simulink model "mrefrobotarm_modified_previous_y_previous_u_previous_ref"  (R2018b)
settings: Solver=FixedStepAuto  StartTime=0.0  StopTime=10  RelTol=1e-3  AbsTol=1e-6
undefined symbols (not defined in the file or in its folder): options, sfunxy2
libraries: neural x949, simulink x1
(part 18 of 31)

== system mrefrobotarm_modified_previous_y_previous_u_previous_ref/const_51traces_100/Layer 2/Delays 1 ==
  "p{2}" : Inport  PortDimensions=100
      mask Display: e = 0.06;c1 = [120 230 180]/255;c2 = ([120 230 180]+0)/(256+128);c3 = ([120 230 180]+128)/(256+128);patch([0 1 1 0],[0 0 1 1],c1);patch([0 1 1 1-e 1-e 0+e],[0 0 1 1-e 0+e 0+e],c2);patch([0 0 1 1-e 0+e 0+e],[0 1 1 1-e 1-e 0+e],c3);plot([0 1 1 0 0],[0 0 1 1 0]);
  mux : Mux  Inputs=1
      mask Display: e = 0.06;c1 = [120 150 230]/255;c2 = ([120 150 230]+0)/383;c3 = ([120 150 230]+128)/383;patch([0 1 1 0],[0 0 1 1],c1);patch([0 1 1 1-e 1-e 0+e],[0 0 1 1-e 0+e 0+e],c2);patch([0 0 1 1-e 0+e 0+e],[0 1 1 1-e 1-e 0+e],c3);plot([0 1 1 0 0],[0 0 1 1 0]);disp('Mux')
  "pd{2,1}" : Outport
      mask Display: e = 0.06;c1 = [120 230 180]/255;c2 = ([120 230 180]+0)/(256+128);c3 = ([120 230 180]+128)/(256+128);patch([0 1 1 0],[0 0 1 1],c1);patch([0 1 1 1-e 1-e 0+e],[0 0 1 1-e 0+e 0+e],c2);patch([0 0 1 1-e 0+e 0+e],[0 1 1 1-e 1-e 0+e],c3);plot([0 1 1 0 0],[0 0 1 1 0]);
  wires:
  "p{2}"/1 -> mux/1
  mux/1 -> "pd{2,1}"/1

== system mrefrobotarm_modified_previous_y_previous_u_previous_ref/const_51traces_100/Layer 2/LW{2,1} ==
  "ad{2,1}" : Inport  PortDimensions=100
      mask Display: e = 0.06;c1 = [120 230 180]/255;c2 = ([120 230 180]+0)/(256+128);c3 = ([120 230 180]+128)/(256+128);patch([0 1 1 0],[0 0 1 1],c1);patch([0 1 1 1-e 1-e 0+e],[0 0 1 1-e 0+e 0+e],c2);patch([0 0 1 1-e 0+e 0+e],[0 1 1 1-e 1-e 0+e],c3);plot([0 1 1 0 0],[0 0 1 1 0]);
  "IW{2,1}(1,:)'" : Constant  Value=[0.0175272454781582980032350604915336589328944683074951171875;0.1037884636130461391001489346308517269790172576904296875;0.1678323451234425556233276211060001514852046966552734375;-0.288603537612614591267856667400337755680084228515625;-0.11505271842033663876048166230248170904815196990966796875;0.484983797057167931310317499082884751260280609130859375;0.6500323943068477827722517758957110345363616943359375;-0.054915350131312955228590766409979551099240779876708984375;0.20376802589153186762160885336925275623798370361328125;0.354036025319482028361761649648542515933513641357421875;0.26383239784267409344664656600798480212688446044921875;-0.4044611855080344486879084797692485153675079345703125;-0.3969973796125929599298842731514014303684234619140625;0.058090970970541187801128302226061350665986537933349609375;0.46097909601718722871765976378810591995716094970703125;0.08145271749453049381362035319398273713886737823486328125;-0.432062703580626372712458760361187160015106201171875;0.0281870579083633270023323547093241359107196331024169921875;-0.2781486542400661843288389718509279191493988037109375;0.352209712985656564487868536161840893328189849853515625;-0.5177328045394247180155389287392608821392059326171875;0.3218612892579877371446173128788359463214874267578125;0.108382262009518226530957463182858191430568695068359375;-0.0281977299513606026459822118113152100704610347747802734375;-0.0222190548546749959413215691483856062404811382293701171875;-0.13714555564807284770978412780095823109149932861328125;0.475820366394926586028901738245622254908084869384765625;-0.2530362662263332396150872227735817432403564453125;1.13592482391357396664943735231645405292510986328125;0.182412512963191664194795293951756320893764495849609375;-0.383173771713362032453886740768211893737316131591796875;0.16752681293786564342696010498912073671817779541015625;0.355499731991164857891618567009572871029376983642578125;-0.472667121504766252204632337452494539320468902587890625;-0.1134559424090527957051932617105194367468357086181640625;0.1431993945862777284361300189630128443241119384765625;-0.34283193773631237544208261169842444360256195068359375;-0.1748292891555640327094778285754728130996227264404296875;0.24866853174265302062195814869483001530170440673828125;-0.0922372121421325685819425643785507418215274810791015625;0.0260131301457378442953949360116894240491092205047607421875;0.53656038287427254562800271742162294685840606689453125;-0.127263729849789009040961218488519079983234405517578125;0.0295598345734353860903009802996166399680078029632568359375;0.06515241877197346098693486737829516641795635223388671875;-0.71592137786966858481463304997305385768413543701171875;0.2145878545350983213069184785126708447933197021484375;0.0174498370969321907331117671446918393485248088836669921875;0.024551444399681772445820371331137721426784992218017578125;-0.0592313819651306971980631033147801645100116729736328125;-0.02656845197032738081777125671578687615692615509033203125;-0.10853440274985927394002516166437999345362186431884765625;0.0966079991763288681294596926818485371768474578857421875;-0.1862460199455625853293128102450282312929630279541015625;0.3522646934737689861094622756354510784149169921875;-0.018777540045504602372883340422049514017999172210693359375;-0.07779695482157784891530383220015210099518299102783203125;-0.51578515564848903540706714920816011726856231689453125;-0.2815557847536551694389572730869986116886138916015625;-0.546587162786270841507985096541233360767364501953125;-0.617119930339165900790021623834036290645599365234375;-0.00426673473403185558872063865010204608552157878875732421875;0.1708548264980287723080465411840123124420642852783203125;-0.1821642425410656962458944008176331408321857452392578125;0.43185805123537723826387946246541105210781097412109375;0.2418901792035169917571835185299278236925601959228515625;0.311021513464165122453408685032627545297145843505859375;0.1609222295496172405737667077119112946093082427978515625;0.10729217408512915776785945354276918806135654449462890625 ...(+1779 chars)]
      mask Display: e = 0.06;c1 = [120 150 230]/255;c2 = ([120 150 230]+0)/383;c3 = ([120 150 230]+128)/383;patch([0 1 1 0],[0 0 1 1],c1);patch([0 1 1 1-e 1-e 0+e],[0 0 1 1-e 0+e 0+e],c2);patch([0 0 1 1-e 0+e 0+e],[0 1 1 1-e 1-e 0+e],c3);plot([0 1 1 0 0],[0 0 1 1 0]);disp('weights');
  Mux : Mux  Inputs=1
      mask Display: e = 0.06;c1 = [120 150 230]/255;c2 = ([120 150 230]+0)/383;c3 = ([120 150 230]+128)/383;patch([0 1 1 0],[0 0 1 1],c1);patch([0 1 1 1-e 1-e 0+e],[0 0 1 1-e 0+e 0+e],c2);patch([0 0 1 1-e 0+e 0+e],[0 1 1 1-e 1-e 0+e],c3);plot([0 1 1 0 0],[0 0 1 1 0]);disp('Mux');
  dotprod1 : neural/Weight Functions/dotprod
  "lz{2,1}" : Outport
      mask Display: e = 0.06;c1 = [120 230 180]/255;c2 = ([120 230 180]+0)/(256+128);c3 = ([120 230 180]+128)/(256+128);patch([0 1 1 0],[0 0 1 1],c1);patch([0 1 1 1-e 1-e 0+e],[0 0 1 1-e 0+e 0+e],c2);patch([0 0 1 1-e 0+e 0+e],[0 1 1 1-e 1-e 0+e],c3);plot([0 1 1 0 0],[0 0 1 1 0]);
  wires:
  "IW{2,1}(1,:)'"/1 -> dotprod1/1
  "ad{2,1}"/1 -> dotprod1/2
  dotprod1/1 -> Mux/1
  Mux/1 -> "lz{2,1}"/1

== system mrefrobotarm_modified_previous_y_previous_u_previous_ref/const_51traces_30x30/Layer 1/Delays 1 ==
  "p{1}" : Inport  PortDimensions=10
      mask Display: e = 0.06;c1 = [120 230 180]/255;c2 = ([120 230 180]+0)/(256+128);c3 = ([120 230 180]+128)/(256+128);patch([0 1 1 0],[0 0 1 1],c1);patch([0 1 1 1-e 1-e 0+e],[0 0 1 1-e 0+e 0+e],c2);patch([0 0 1 1-e 0+e 0+e],[0 1 1 1-e 1-e 0+e],c3);plot([0 1 1 0 0],[0 0 1 1 0]);
  mux : Mux  Inputs=1
      mask Display: e = 0.06;c1 = [120 150 230]/255;c2 = ([120 150 230]+0)/383;c3 = ([120 150 230]+128)/383;patch([0 1 1 0],[0 0 1 1],c1);patch([0 1 1 1-e 1-e 0+e],[0 0 1 1-e 0+e 0+e],c2);patch([0 0 1 1-e 0+e 0+e],[0 1 1 1-e 1-e 0+e],c3);plot([0 1 1 0 0],[0 0 1 1 0]);disp('Mux')
  "pd{1,1}" : Outport
      mask Display: e = 0.06;c1 = [120 230 180]/255;c2 = ([120 230 180]+0)/(256+128);c3 = ([120 230 180]+128)/(256+128);patch([0 1 1 0],[0 0 1 1],c1);patch([0 1 1 1-e 1-e 0+e],[0 0 1 1-e 0+e 0+e],c2);patch([0 0 1 1-e 0+e 0+e],[0 1 1 1-e 1-e 0+e],c3);plot([0 1 1 0 0],[0 0 1 1 0]);
  wires:
  "p{1}"/1 -> mux/1
  mux/1 -> "pd{1,1}"/1

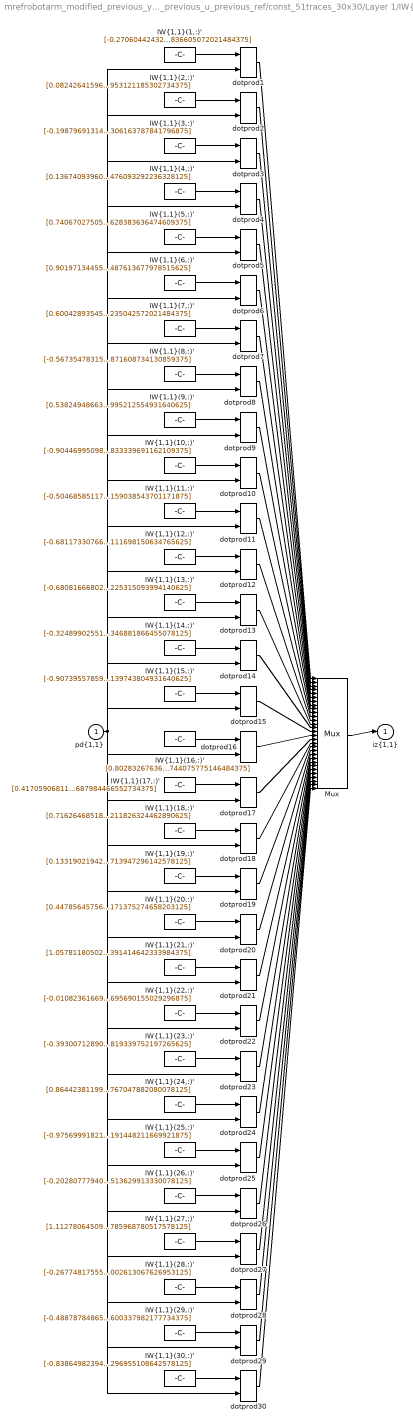
== system mrefrobotarm_modified_previous_y_previous_u_previous_ref/const_51traces_30x30/Layer 1/IW{1,1} ==
  "pd{1,1}" : Inport  PortDimensions=10
      mask Display: e = 0.06;c1 = [120 230 180]/255;c2 = ([120 230 180]+0)/(256+128);c3 = ([120 230 180]+128)/(256+128);patch([0 1 1 0],[0 0 1 1],c1);patch([0 1 1 1-e 1-e 0+e],[0 0 1 1-e 0+e 0+e],c2);patch([0 0 1 1-e 0+e 0+e],[0 1 1 1-e 1-e 0+e],c3);plot([0 1 1 0 0],[0 0 1 1 0]);
  "IW{1,1}(1,:)'" : Constant  Value=[-0.270604424325050108013357430536416359245777130126953125;0.70004440133500034360025665591820143163204193115234375;-0.70617231900424692891959921325906179845333099365234375;0.74614133159121009963854476154665462672710418701171875;-0.305217301709377719642901638508192263543605804443359375;0.319535451212445475999146538015338592231273651123046875;0.621085602068974562683933982043527066707611083984375;0.63854127804799520884415642285603098571300506591796875;-0.5262324480762945455580847919918596744537353515625;0.58139367724695334427309489910840056836605072021484375]
      mask Display: e = 0.06;c1 = [120 150 230]/255;c2 = ([120 150 230]+0)/383;c3 = ([120 150 230]+128)/383;patch([0 1 1 0],[0 0 1 1],c1);patch([0 1 1 1-e 1-e 0+e],[0 0 1 1-e 0+e 0+e],c2);patch([0 0 1 1-e 0+e 0+e],[0 1 1 1-e 1-e 0+e],c3);plot([0 1 1 0 0],[0 0 1 1 0]);disp('Weights');
  "IW{1,1}(10,:)'" : Constant  Value=[-0.904469950985906212537202009116299450397491455078125;0.0053775612000614599061965037662957911379635334014892578125;0.36226460789501124803990705913747660815715789794921875;0.61558596620200811688761177720152772963047027587890625;-0.771838905191784885317929365555755794048309326171875;0.41100345723550313348226836751564405858516693115234375;0.99775813612685648745781463730963878333568572998046875;-0.7258966477236088454816353987553156912326812744140625;0.339809360766077428461784393221023492515087127685546875;-0.374697354634937251915971501148305833339691162109375]
      mask Display: e = 0.06;c1 = [120 150 230]/255;c2 = ([120 150 230]+0)/383;c3 = ([120 150 230]+128)/383;patch([0 1 1 0],[0 0 1 1],c1);patch([0 1 1 1-e 1-e 0+e],[0 0 1 1-e 0+e 0+e],c2);patch([0 0 1 1-e 0+e 0+e],[0 1 1 1-e 1-e 0+e],c3);plot([0 1 1 0 0],[0 0 1 1 0]);disp('Weights');
  "IW{1,1}(11,:)'" : Constant  Value=[-0.50468585117887254654078788007609546184539794921875;-0.68954953293469911645985348513931967318058013916015625;-0.66542598505421379773139278768212534487247467041015625;0.2389505818090202904357965962844900786876678466796875;-0.9069520006432707504018253530375659465789794921875;-0.00929102406457815895024499042165189166553318500518798828125;-0.080408409383206258524978693458251655101776123046875;-0.0307560022462756814387585535541802528314292430877685546875;-0.5095518302180745973117836911114864051342010498046875;-0.1912185596962409916965697220803122036159038543701171875]
      mask Display: e = 0.06;c1 = [120 150 230]/255;c2 = ([120 150 230]+0)/383;c3 = ([120 150 230]+128)/383;patch([0 1 1 0],[0 0 1 1],c1);patch([0 1 1 1-e 1-e 0+e],[0 0 1 1-e 0+e 0+e],c2);patch([0 0 1 1-e 0+e 0+e],[0 1 1 1-e 1-e 0+e],c3);plot([0 1 1 0 0],[0 0 1 1 0]);disp('Weights');
  "IW{1,1}(12,:)'" : Constant  Value=[-0.6811733076649948426251057753688655793666839599609375;0.767168777444947824761811716598458588123321533203125;-0.83256168597038582301905762506066821515560150146484375;0.349181571891764408466229951955028809607028961181640625;-0.3909137437032808026771135700982995331287384033203125;0.793416678289866172946176448022015392780303955078125;-0.26568946573439500280500169537845067679882049560546875;0.31350215743328291306823984996299259364604949951171875;0.54821743072928519335818009494687430560588836669921875;0.32038657144986493197080790196196176111698150634765625]
      mask Display: e = 0.06;c1 = [120 150 230]/255;c2 = ([120 150 230]+0)/383;c3 = ([120 150 230]+128)/383;patch([0 1 1 0],[0 0 1 1],c1);patch([0 1 1 1-e 1-e 0+e],[0 0 1 1-e 0+e 0+e],c2);patch([0 0 1 1-e 0+e 0+e],[0 1 1 1-e 1-e 0+e],c3);plot([0 1 1 0 0],[0 0 1 1 0]);disp('Weights');
  "IW{1,1}(13,:)'" : Constant  Value=[-0.68081666802457185827535113276098854839801788330078125;-0.401968341120073180405825041816569864749908447265625;-0.742671527584819468614796278416179120540618896484375;0.55481882178189090293329854830517433583736419677734375;-0.10552588707788358723949073691983358003199100494384765625;0.637373365340767605857763555832207202911376953125;-0.8353233744383405934286201954819262027740478515625;-0.29899770642931267072839318643673323094844818115234375;0.564632412351024459695736368303187191486358642578125;0.7292360747751518434967010762193240225315093994140625]
      mask Display: e = 0.06;c1 = [120 150 230]/255;c2 = ([120 150 230]+0)/383;c3 = ([120 150 230]+128)/383;patch([0 1 1 0],[0 0 1 1],c1);patch([0 1 1 1-e 1-e 0+e],[0 0 1 1-e 0+e 0+e],c2);patch([0 0 1 1-e 0+e 0+e],[0 1 1 1-e 1-e 0+e],c3);plot([0 1 1 0 0],[0 0 1 1 0]);disp('Weights');
  "IW{1,1}(14,:)'" : Constant  Value=[-0.3248990255155626005745261863921768963336944580078125;0.76936888369251799080217324444674886763095855712890625;0.25362880157654610346895651673548854887485504150390625;-0.385148254088853281285054208638030104339122772216796875;0.903008203587827740221882777404971420764923095703125;-0.86201801339850447902790619991719722747802734375;-0.03766018743441447436115510072340839542448520660400390625;-0.2495959672245479377128418718712055124342441558837890625;0.4682185834363934429092068967293016612529754638671875;-0.150318483037516437139657909938250668346881866455078125]
      mask Display: e = 0.06;c1 = [120 150 230]/255;c2 = ([120 150 230]+0)/383;c3 = ([120 150 230]+128)/383;patch([0 1 1 0],[0 0 1 1],c1);patch([0 1 1 1-e 1-e 0+e],[0 0 1 1-e 0+e 0+e],c2);patch([0 0 1 1-e 0+e 0+e],[0 1 1 1-e 1-e 0+e],c3);plot([0 1 1 0 0],[0 0 1 1 0]);disp('Weights');
  "IW{1,1}(15,:)'" : Constant  Value=[-0.907395578595841190150395050295628607273101806640625;-0.30512097353865808013750893223914317786693572998046875;0.5828010439283024535228605600423179566860198974609375;0.31263263801523144547189758668537251651287078857421875;-0.57075352243817822905924685983336530625820159912109375;-0.849041027833965955551320803351700305938720703125;-0.1980749653500880336221001698504551313817501068115234375;0.5771746804102126926494520375854335725307464599609375;-0.8655995602268304889292949155787937343120574951171875;-0.455835103623935256056398657165118493139743804931640625]
      mask Display: e = 0.06;c1 = [120 150 230]/255;c2 = ([120 150 230]+0)/383;c3 = ([120 150 230]+128)/383;patch([0 1 1 0],[0 0 1 1],c1);patch([0 1 1 1-e 1-e 0+e],[0 0 1 1-e 0+e 0+e],c2);patch([0 0 1 1-e 0+e 0+e],[0 1 1 1-e 1-e 0+e],c3);plot([0 1 1 0 0],[0 0 1 1 0]);disp('Weights');
  "IW{1,1}(16,:)'" : Constant  Value=[0.8028326763653514941410094252205453813076019287109375;0.2135282302308567914383985453241621144115924835205078125;-0.53658547925477606543864794730325229465961456298828125;-0.58436633746776944775547235622070729732513427734375;0.58594054556996300053839377142139710485935211181640625;0.52944330814025153397750500516849569976329803466796875;0.5813357493280018051251545330160297453403472900390625;0.0542018352808505132767180612063384614884853363037109375;-0.49630452081610532122368795171496458351612091064453125;0.51756102414473603712252725017606280744075775146484375]
      mask Display: e = 0.06;c1 = [120 150 230]/255;c2 = ([120 150 230]+0)/383;c3 = ([120 150 230]+128)/383;patch([0 1 1 0],[0 0 1 1],c1);patch([0 1 1 1-e 1-e 0+e],[0 0 1 1-e 0+e 0+e],c2);patch([0 0 1 1-e 0+e 0+e],[0 1 1 1-e 1-e 0+e],c3);plot([0 1 1 0 0],[0 0 1 1 0]);disp('Weights');
  "IW{1,1}(17,:)'" : Constant  Value=[0.417059068118903419897236517499550245702266693115234375;0.86693872973463736997246087412349879741668701171875;-0.09736053006628204997685571697729756124317646026611328125;-0.26652183644718052679678521599271334707736968994140625;-0.78527287431403058892698254567221738398075103759765625;0.72331509355932244176301537663675844669342041015625;-0.499391660010226112742515169884427450597286224365234375;-0.2005656034671676468672529836112516932189464569091796875;0.484066919932689077032961222357698716223239898681640625;-0.3797347694610289092764787710621021687984466552734375]
      mask Display: e = 0.06;c1 = [120 150 230]/255;c2 = ([120 150 230]+0)/383;c3 = ([120 150 230]+128)/383;patch([0 1 1 0],[0 0 1 1],c1);patch([0 1 1 1-e 1-e 0+e],[0 0 1 1-e 0+e 0+e],c2);patch([0 0 1 1-e 0+e 0+e],[0 1 1 1-e 1-e 0+e],c3);plot([0 1 1 0 0],[0 0 1 1 0]);disp('Weights');
  "IW{1,1}(18,:)'" : Constant  Value=[0.71626468518987085332128117443062365055084228515625;-0.8876691191192678243027103235363028943538665771484375;0.039176884968088181160350558229765738360583782196044921875;0.499624896919878935808156938946922309696674346923828125;0.66300864191458386276423198069096542894840240478515625;-0.87515620412197858701830455174786038696765899658203125;-0.1514988063602618895142626342931180261075496673583984375;-0.0930009582912652288388954957554233260452747344970703125;0.240872117926244910801614196316222660243511199951171875;-0.5643150519818969090835025781416334211826324462890625]
      mask Display: e = 0.06;c1 = [120 150 230]/255;c2 = ([120 150 230]+0)/383;c3 = ([120 150 230]+128)/383;patch([0 1 1 0],[0 0 1 1],c1);patch([0 1 1 1-e 1-e 0+e],[0 0 1 1-e 0+e 0+e],c2);patch([0 0 1 1-e 0+e 0+e],[0 1 1 1-e 1-e 0+e],c3);plot([0 1 1 0 0],[0 0 1 1 0]);disp('Weights');
  "IW{1,1}(19,:)'" : Constant  Value=[0.1331902194200601796669758414282114244997501373291015625;-1.206531645099333527326734838425181806087493896484375;-0.2034788121763428658805850091084721498191356658935546875;0.75158830964644562921961323809227906167507171630859375;0.2168916980824796281179800416794023476541042327880859375;0.95211063189393740913146757520735263824462890625;-0.14342326109423897406713876989670097827911376953125;-0.331154788610227956979770169709809124469757080078125;0.48262930350819022162767168993013910949230194091796875;0.6904149972961513004321432163123972713947296142578125]
      mask Display: e = 0.06;c1 = [120 150 230]/255;c2 = ([120 150 230]+0)/383;c3 = ([120 150 230]+128)/383;patch([0 1 1 0],[0 0 1 1],c1);patch([0 1 1 1-e 1-e 0+e],[0 0 1 1-e 0+e 0+e],c2);patch([0 0 1 1-e 0+e 0+e],[0 1 1 1-e 1-e 0+e],c3);plot([0 1 1 0 0],[0 0 1 1 0]);disp('Weights');
  "IW{1,1}(2,:)'" : Constant  Value=[0.08242641596592147068545131105565815232694149017333984375;-0.63132380330906368026688824102166108787059783935546875;-0.42419128375723313961742633182439021766185760498046875;-0.349541913136007298401608522908645682036876678466796875;0.3955394556467781708164466181187890470027923583984375;-0.1608872230926843560627759188719210214912891387939453125;-0.64645796976916736209517466704710386693477630615234375;0.162461414513925761493595700812875293195247650146484375;-0.9431839182811787569704620182164944708347320556640625;0.88701558171751082593203818760230205953121185302734375]
      mask Display: e = 0.06;c1 = [120 150 230]/255;c2 = ([120 150 230]+0)/383;c3 = ([120 150 230]+128)/383;patch([0 1 1 0],[0 0 1 1],c1);patch([0 1 1 1-e 1-e 0+e],[0 0 1 1-e 0+e 0+e],c2);patch([0 0 1 1-e 0+e 0+e],[0 1 1 1-e 1-e 0+e],c3);plot([0 1 1 0 0],[0 0 1 1 0]);disp('Weights');
  "IW{1,1}(20,:)'" : Constant  Value=[0.4478564575662946634082572927582077682018280029296875;-1.222475833910656728420462968642823398113250732421875;0.79118610964665148088670321158133447170257568359375;-0.10684286029015420405041680851354612968862056732177734375;0.73918884559817221724387081849272362887859344482421875;0.011971039641693541344391604752672719769179821014404296875;0.416590194532186763876069335310603491961956024169921875;-0.04977109102469097490217819768076878972351551055908203125;0.09644638024768890927074238561544916592538356781005859375;0.70696142605753220511388690283638425171375274658203125]
      mask Display: e = 0.06;c1 = [120 150 230]/255;c2 = ([120 150 230]+0)/383;c3 = ([120 150 230]+128)/383;patch([0 1 1 0],[0 0 1 1],c1);patch([0 1 1 1-e 1-e 0+e],[0 0 1 1-e 0+e 0+e],c2);patch([0 0 1 1-e 0+e 0+e],[0 1 1 1-e 1-e 0+e],c3);plot([0 1 1 0 0],[0 0 1 1 0]);disp('Weights');
  "IW{1,1}(21,:)'" : Constant  Value=[1.05781180502420024680532151251100003719329833984375;0.03122644943323150956704381542294868268072605133056640625;0.50586496692193627655598220371757633984088897705078125;-0.9237102161489689766682431582012213766574859619140625;-0.87152798298566647172691546074929647147655487060546875;0.72217289797899930636759791013901121914386749267578125;-0.93970244549850601156748552966746501624584197998046875;0.09951791143973587328019902997766621410846710205078125;-0.07916119208580559007959465134263155050575733184814453125;-0.2391904909273630808197452779495506547391414642333984375]
      mask Display: e = 0.06;c1 = [120 150 230]/255;c2 = ([120 150 230]+0)/383;c3 = ([120 150 230]+128)/383;patch([0 1 1 0],[0 0 1 1],c1);patch([0 1 1 1-e 1-e 0+e],[0 0 1 1-e 0+e 0+e],c2);patch([0 0 1 1-e 0+e 0+e],[0 1 1 1-e 1-e 0+e],c3);plot([0 1 1 0 0],[0 0 1 1 0]);disp('Weights');
  "IW{1,1}(22,:)'" : Constant  Value=[-0.01082361669861600823872027632432946120388805866241455078125;0.258843638292018785040937700614449568092823028564453125;-0.2732784088971051961181046863202936947345733642578125;0.46883652356743976685748975796741433441638946533203125;0.061236281133378651919674240389213082380592823028564453125;0.262077975615905567341457071961485780775547027587890625;1.111616118766455496569278693641535937786102294921875;0.56521150012436305321017471214872784912586212158203125;0.283215405086767957332227751976461149752140045166015625;0.603760442760037374654302766430191695690155029296875]
      mask Display: e = 0.06;c1 = [120 150 230]/255;c2 = ([120 150 230]+0)/383;c3 = ([120 150 230]+128)/383;patch([0 1 1 0],[0 0 1 1],c1);patch([0 1 1 1-e 1-e 0+e],[0 0 1 1-e 0+e 0+e],c2);patch([0 0 1 1-e 0+e 0+e],[0 1 1 1-e 1-e 0+e],c3);plot([0 1 1 0 0],[0 0 1 1 0]);disp('Weights');
  "IW{1,1}(23,:)'" : Constant  Value=[-0.39300712890868705340352562416228465735912322998046875;-0.69258702889495304955147503278567455708980560302734375;-0.373921978919962427756473744011600501835346221923828125;0.93556853200473788501057015309925191104412078857421875;-0.15652755210370383753826217798632569611072540283203125;0.636759646882385954569372188416309654712677001953125;-0.71703138317757708630750812517362646758556365966796875;-0.74749736264166255494956203619949519634246826171875;0.61427400438070633992282409963081590831279754638671875;0.246264245345828192146342416890547610819339752197265625]
      mask Display: e = 0.06;c1 = [120 150 230]/255;c2 = ([120 150 230]+0)/383;c3 = ([120 150 230]+128)/383;patch([0 1 1 0],[0 0 1 1],c1);patch([0 1 1 1-e 1-e 0+e],[0 0 1 1-e 0+e 0+e],c2);patch([0 0 1 1-e 0+e 0+e],[0 1 1 1-e 1-e 0+e],c3);plot([0 1 1 0 0],[0 0 1 1 0]);disp('Weights');
  "IW{1,1}(24,:)'" : Constant  Value=[0.8644238119931932917694439311162568628787994384765625;0.34093480459637459656363489557406865060329437255859375;0.371427477344157985772454821926658041775226593017578125;-0.2407333661613509645516018053967854939401149749755859375;-0.76178643060511797013845125547959469258785247802734375;0.86249621155050359977423113377881236374378204345703125;-0.136409437374599151748810754725127480924129486083984375;0.7463481418502346809162872887100093066692352294921875;0.1184113939616398825105392234036116860806941986083984375;-0.187912142343233334873531248376821167767047882080078125]
      mask Display: e = 0.06;c1 = [120 150 230]/255;c2 = ([120 150 230]+0)/383;c3 = ([120 150 230]+128)/383;patch([0 1 1 0],[0 0 1 1],c1);patch([0 1 1 1-e 1-e 0+e],[0 0 1 1-e 0+e 0+e],c2);patch([0 0 1 1-e 0+e 0+e],[0 1 1 1-e 1-e 0+e],c3);plot([0 1 1 0 0],[0 0 1 1 0]);disp('Weights');
  "IW{1,1}(25,:)'" : Constant  Value=[-0.97569991821397017428552089768345467746257781982421875;-0.07897013491161607168233871334450668655335903167724609375;0.86163425113067215743711813047411851584911346435546875;0.87202722984251612725614677401608787477016448974609375;0.01326554761724424609525829765743765165098011493682861328125;-0.189894253504417964695250020668026991188526153564453125;-1.0108588342975310947480238610296510159969329833984375;0.382086017042396031140327750108554027974605560302734375;-0.06073083026854865507093705900842905975878238677978515625;-0.047426031656457805218973788896619225852191448211669921875]
      mask Display: e = 0.06;c1 = [120 150 230]/255;c2 = ([120 150 230]+0)/383;c3 = ([120 150 230]+128)/383;patch([0 1 1 0],[0 0 1 1],c1);patch([0 1 1 1-e 1-e 0+e],[0 0 1 1-e 0+e 0+e],c2);patch([0 0 1 1-e 0+e 0+e],[0 1 1 1-e 1-e 0+e],c3);plot([0 1 1 0 0],[0 0 1 1 0]);disp('Weights');
  "IW{1,1}(26,:)'" : Constant  Value=[-0.2028077794078876616712392433328204788267612457275390625;-0.60561867284921977461209507964667864143848419189453125;0.399636491474315291849705999993602745234966278076171875;-0.570451491590937553866069720243103802204132080078125;0.3361090096534684601436993034440092742443084716796875;-0.92774459892175020758742221005377359688282012939453125;0.41770599866879276618192307068966329097747802734375;-0.89373875880271003158128451104857958853244781494140625;-0.165929890307822514028401883479091338813304901123046875;0.61322158559554929002644030333613045513629913330078125]
      mask Display: e = 0.06;c1 = [120 150 230]/255;c2 = ([120 150 230]+0)/383;c3 = ([120 150 230]+128)/383;patch([0 1 1 0],[0 0 1 1],c1);patch([0 1 1 1-e 1-e 0+e],[0 0 1 1-e 0+e 0+e],c2);patch([0 0 1 1-e 0+e 0+e],[0 1 1 1-e 1-e 0+e],c3);plot([0 1 1 0 0],[0 0 1 1 0]);disp('Weights');
  "IW{1,1}(27,:)'" : Constant  Value=[1.112780645095628795360198637354187667369842529296875;-0.6964367858267006550221367433550767600536346435546875;0.00884965519431458839949566907989719766192138195037841796875;-0.61273903040461241698011463086004368960857391357421875;-0.6264796257408249413600742627750150859355926513671875;0.3860913834735975047607325905119068920612335205078125;0.319904529376099311388514934151316992938518524169921875;0.6038797039650922737763494296814315021038055419921875;0.2370247733775322218630066117839305661618709564208984375;-0.55138013522019158063613986087148077785968780517578125]
      mask Display: e = 0.06;c1 = [120 150 230]/255;c2 = ([120 150 230]+0)/383;c3 = ([120 150 230]+128)/383;patch([0 1 1 0],[0 0 1 1],c1);patch([0 1 1 1-e 1-e 0+e],[0 0 1 1-e 0+e 0+e],c2);patch([0 0 1 1-e 0+e 0+e],[0 1 1 1-e 1-e 0+e],c3);plot([0 1 1 0 0],[0 0 1 1 0]);disp('Weights');
  "IW{1,1}(28,:)'" : Constant  Value=[-0.267748175553851164298890807913267053663730621337890625;-0.79570680794114057032828668525326065719127655029296875;0.987345385617238502362624785746447741985321044921875;-0.56480031263848518019443645243882201611995697021484375;0.050331909881582682919631821505390689708292484283447265625;-0.353794920756195174771363554100389592349529266357421875;-0.56948061340765854243528565348242409527301788330078125;-0.52399164791863983570152640822925604879856109619140625;-0.09961386826591585308410259358424809761345386505126953125;-0.5464270550541669990707305260002613067626953125]
      mask Display: e = 0.06;c1 = [120 150 230]/255;c2 = ([120 150 230]+0)/383;c3 = ([120 150 230]+128)/383;patch([0 1 1 0],[0 0 1 1],c1);patch([0 1 1 1-e 1-e 0+e],[0 0 1 1-e 0+e 0+e],c2);patch([0 0 1 1-e 0+e 0+e],[0 1 1 1-e 1-e 0+e],c3);plot([0 1 1 0 0],[0 0 1 1 0]);disp('Weights');
  "IW{1,1}(29,:)'" : Constant  Value=[-0.488787848657793178031027991892187856137752532958984375;0.68073229203107066265232560908771120011806488037109375;-0.61585293106328642398494821463827975094318389892578125;-0.3055877787781844379111362286494113504886627197265625;0.86006364569680326948031279243878088891506195068359375;0.771418393493718657083491052617318928241729736328125;0.308434168123604190991926543574663810431957244873046875;0.2159797683612250385198905178185668773949146270751953125;0.11351479083448356988128580269403755664825439453125;0.224754874030561546671691530718817375600337982177734375]
      mask Display: e = 0.06;c1 = [120 150 230]/255;c2 = ([120 150 230]+0)/383;c3 = ([120 150 230]+128)/383;patch([0 1 1 0],[0 0 1 1],c1);patch([0 1 1 1-e 1-e 0+e],[0 0 1 1-e 0+e 0+e],c2);patch([0 0 1 1-e 0+e 0+e],[0 1 1 1-e 1-e 0+e],c3);plot([0 1 1 0 0],[0 0 1 1 0]);disp('Weights');
  "IW{1,1}(3,:)'" : Constant  Value=[-0.198796913147241183228430827512056566774845123291015625;-0.08673180668299958206990396547553245909512042999267578125;-0.52972817481244238724258366346475668251514434814453125;-0.2464505557089952947347200051808613352477550506591796875;-0.66720002033756731218971935959416441619396209716796875;-0.77504002216581391326855055012856610119342803955078125;-0.5176994856900309915914704106398858129978179931640625;0.83816664325644152366834305212250910699367523193359375;0.5793502590473094127077047232887707650661468505859375;0.64372600748133368409042986968415789306163787841796875]
      mask Display: e = 0.06;c1 = [120 150 230]/255;c2 = ([120 150 230]+0)/383;c3 = ([120 150 230]+128)/383;patch([0 1 1 0],[0 0 1 1],c1);patch([0 1 1 1-e 1-e 0+e],[0 0 1 1-e 0+e 0+e],c2);patch([0 0 1 1-e 0+e 0+e],[0 1 1 1-e 1-e 0+e],c3);plot([0 1 1 0 0],[0 0 1 1 0]);disp('Weights');
  "IW{1,1}(30,:)'" : Constant  Value=[-0.8386498239454238667889285352430306375026702880859375;-0.8904035836865793474004249219433404505252838134765625;0.340726768590182971241375753379543311893939971923828125;-0.00193876221280711471921243127525258387322537600994110107421875;-0.030187288477159394950444237792908097617328166961669921875;-0.300728992270598405323056567794992588460445404052734375;0.1737743130397286506205745126862893812358379364013671875;0.032725490754728338294032852218151674605906009674072265625;0.97125921814589144531737474608235061168670654296875;0.26509745411311691487554753621225245296955108642578125]
      mask Display: e = 0.06;c1 = [120 150 230]/255;c2 = ([120 150 230]+0)/383;c3 = ([120 150 230]+128)/383;patch([0 1 1 0],[0 0 1 1],c1);patch([0 1 1 1-e 1-e 0+e],[0 0 1 1-e 0+e 0+e],c2);patch([0 0 1 1-e 0+e 0+e],[0 1 1 1-e 1-e 0+e],c3);plot([0 1 1 0 0],[0 0 1 1 0]);disp('Weights');
  "IW{1,1}(4,:)'" : Constant  Value=[0.1367409396095775886426082479374599643051624298095703125;0.63333776924836604482749180533573962748050689697265625;0.433875938172473663012596034604939632117748260498046875;0.63840157530002539232327762874774634838104248046875;-0.227328653834083016516132147444295696914196014404296875;-0.44556948935937279454577719661756418645381927490234375;0.67209785173148561820966051527648232877254486083984375;-0.166710736440739470953786849349853582680225372314453125;0.472497710885404098579698484172695316374301910400390625;0.49082263915346857618970943804015405476093292236328125]
      mask Display: e = 0.06;c1 = [120 150 230]/255;c2 = ([120 150 230]+0)/383;c3 = ([120 150 230]+128)/383;patch([0 1 1 0],[0 0 1 1],c1);patch([0 1 1 1-e 1-e 0+e],[0 0 1 1-e 0+e 0+e],c2);patch([0 0 1 1-e 0+e 0+e],[0 1 1 1-e 1-e 0+e],c3);plot([0 1 1 0 0],[0 0 1 1 0]);disp('Weights');
  "IW{1,1}(5,:)'" : Constant  Value=[0.7406702750530602674672309149173088371753692626953125;-0.022721491821038407310506812564199208281934261322021484375;0.284673294546059774123847319060587324202060699462890625;-0.86462954394894786513958706564153544604778289794921875;-0.37048866930498991489884019756573252379894256591796875;0.507520243202882692656885410542599856853485107421875;-0.839236511131892459758319091633893549442291259765625;-0.227924994350555021327409122022800147533416748046875;-0.149286962017158353344115084837540052831172943115234375;-0.99865305624165667808256330317817628383636474609375]
      mask Display: e = 0.06;c1 = [120 150 230]/255;c2 = ([120 150 230]+0)/383;c3 = ([120 150 230]+128)/383;patch([0 1 1 0],[0 0 1 1],c1);patch([0 1 1 1-e 1-e 0+e],[0 0 1 1-e 0+e 0+e],c2);patch([0 0 1 1-e 0+e 0+e],[0 1 1 1-e 1-e 0+e],c3);plot([0 1 1 0 0],[0 0 1 1 0]);disp('Weights');
  "IW{1,1}(6,:)'" : Constant  Value=[0.9019713445568964260701250168494880199432373046875;0.2578434447365653969796994715579785406589508056640625;0.513439679192137621299707461730577051639556884765625;-0.4570290205027995877884450237615965306758880615234375;-0.420389646693099139351801341035752557218074798583984375;-0.345864414796718311340129048403468914330005645751953125;0.349335382152383966403164095027022995054721832275390625;-0.10395800942993500826094788180853356607258319854736328125;-0.9451530926156495038270577424555085599422454833984375;-1.19982929853263531327911550761200487613677978515625]
      mask Display: e = 0.06;c1 = [120 150 230]/255;c2 = ([120 150 230]+0)/383;c3 = ([120 150 230]+128)/383;patch([0 1 1 0],[0 0 1 1],c1);patch([0 1 1 1-e 1-e 0+e],[0 0 1 1-e 0+e 0+e],c2);patch([0 0 1 1-e 0+e 0+e],[0 1 1 1-e 1-e 0+e],c3);plot([0 1 1 0 0],[0 0 1 1 0]);disp('Weights');
  "IW{1,1}(7,:)'" : Constant  Value=[0.60042893545997666482350041405879892408847808837890625;0.186376878960270442320279471459798514842987060546875;0.401135546163025991095452127410680986940860748291015625;0.2534309058297334882325912985834293067455291748046875;-0.9079555993883545728095896265585906803607940673828125;-0.800112944617791921331217963597737252712249755859375;0.71442567942073187392537647610879503190517425537109375;-0.376216353261814850927891029641614295542240142822265625;0.2115831704254899359174402206917875446379184722900390625;-0.8563889303715954692819423144101165235042572021484375]
      mask Display: e = 0.06;c1 = [120 150 230]/255;c2 = ([120 150 230]+0)/383;c3 = ([120 150 230]+128)/383;patch([0 1 1 0],[0 0 1 1],c1);patch([0 1 1 1-e 1-e 0+e],[0 0 1 1-e 0+e 0+e],c2);patch([0 0 1 1-e 0+e 0+e],[0 1 1 1-e 1-e 0+e],c3);plot([0 1 1 0 0],[0 0 1 1 0]);disp('Weights');
  "IW{1,1}(8,:)'" : Constant  Value=[-0.567354783153465103140433711814694106578826904296875;0.65100653848125944467284398342599160969257354736328125;-0.08763341420107477464096490393785643391311168670654296875;-0.696514537154315771516621680348180234432220458984375;0.278384438128423450375947822976741008460521697998046875;-0.1874317061257641248150918045212165452539920806884765625;-0.1579570062114115380769163721197401173412799835205078125;1.046683553063931793047913743066601455211639404296875;-0.61546267705748503029639095984748564660549163818359375;-0.7688370194155762504806261858902871608734130859375]
      mask Display: e = 0.06;c1 = [120 150 230]/255;c2 = ([120 150 230]+0)/383;c3 = ([120 150 230]+128)/383;patch([0 1 1 0],[0 0 1 1],c1);patch([0 1 1 1-e 1-e 0+e],[0 0 1 1-e 0+e 0+e],c2);patch([0 0 1 1-e 0+e 0+e],[0 1 1 1-e 1-e 0+e],c3);plot([0 1 1 0 0],[0 0 1 1 0]);disp('Weights');
  "IW{1,1}(9,:)'" : Constant  Value=[0.53824948663072458288070265552960336208343505859375;-1.038240524192894920219032428576610982418060302734375;-0.324359970368811811880505047156475484371185302734375;0.4139735971084821386511976015754044055938720703125;-0.492876926015802296898726808649371378123760223388671875;-0.310918531349678506359168750350363552570343017578125;-0.277665784878947885516708993236534297466278076171875;-0.07967083872044511405619005017797462642192840576171875;0.418656489643839890835153028092463500797748565673828125;-1.121737015202770582078528605052269995212554931640625]
      mask Display: e = 0.06;c1 = [120 150 230]/255;c2 = ([120 150 230]+0)/383;c3 = ([120 150 230]+128)/383;patch([0 1 1 0],[0 0 1 1],c1);patch([0 1 1 1-e 1-e 0+e],[0 0 1 1-e 0+e 0+e],c2);patch([0 0 1 1-e 0+e 0+e],[0 1 1 1-e 1-e 0+e],c3);plot([0 1 1 0 0],[0 0 1 1 0]);disp('Weights');
  Mux : Mux  Inputs=30
      mask Display: e = 0.06;c1 = [120 150 230]/255;c2 = ([120 150 230]+0)/383;c3 = ([120 150 230]+128)/383;patch([0 1 1 0],[0 0 1 1],c1);patch([0 1 1 1-e 1-e 0+e],[0 0 1 1-e 0+e 0+e],c2);patch([0 0 1 1-e 0+e 0+e],[0 1 1 1-e 1-e 0+e],c3);plot([0 1 1 0 0],[0 0 1 1 0]);disp('Mux');
  dotprod{1..30} (30 alike) : neural/Weight Functions/dotprod
  "iz{1,1}" : Outport
      mask Display: e = 0.06;c1 = [120 230 180]/255;c2 = ([120 230 180]+0)/(256+128);c3 = ([120 230 180]+128)/(256+128);patch([0 1 1 0],[0 0 1 1],c1);patch([0 1 1 1-e 1-e 0+e],[0 0 1 1-e 0+e 0+e],c2);patch([0 0 1 1-e 0+e 0+e],[0 1 1 1-e 1-e 0+e],c3);plot([0 1 1 0 0],[0 0 1 1 0]);
  wires:
  "IW{1,1}(1,:)'"/1 -> dotprod1/1
  "pd{1,1}"/1 -> dotprod1/2, dotprod2/2, dotprod3/2, dotprod4/2, dotprod5/2, dotprod6/2, dotprod7/2, dotprod8/2, dotprod9/2, dotprod10/2, dotprod11/2, dotprod12/2, dotprod13/2, dotprod14/2, dotprod15/2, dotprod16/2, dotprod17/2, dotprod18/2, dotprod19/2, dotprod20/2, dotprod21/2, dotprod22/2, dotprod23/2, dotprod24/2, dotprod25/2, dotprod26/2, dotprod27/2, dotprod28/2, dotprod29/2, dotprod30/2
  dotprod1/1 -> Mux/1
  "IW{1,1}(2,:)'"/1 -> dotprod2/1
  dotprod2/1 -> Mux/2
  "IW{1,1}(3,:)'"/1 -> dotprod3/1
  dotprod3/1 -> Mux/3
  "IW{1,1}(4,:)'"/1 -> dotprod4/1
  dotprod4/1 -> Mux/4
  "IW{1,1}(5,:)'"/1 -> dotprod5/1
  dotprod5/1 -> Mux/5
  "IW{1,1}(6,:)'"/1 -> dotprod6/1
  dotprod6/1 -> Mux/6
  "IW{1,1}(7,:)'"/1 -> dotprod7/1
  dotprod7/1 -> Mux/7
  "IW{1,1}(8,:)'"/1 -> dotprod8/1
  dotprod8/1 -> Mux/8
  "IW{1,1}(9,:)'"/1 -> dotprod9/1
  dotprod9/1 -> Mux/9
  "IW{1,1}(10,:)'"/1 -> dotprod10/1
  dotprod10/1 -> Mux/10
  "IW{1,1}(11,:)'"/1 -> dotprod11/1
  dotprod11/1 -> Mux/11
  "IW{1,1}(12,:)'"/1 -> dotprod12/1
  dotprod12/1 -> Mux/12
  "IW{1,1}(13,:)'"/1 -> dotprod13/1
  dotprod13/1 -> Mux/13
  "IW{1,1}(14,:)'"/1 -> dotprod14/1
  dotprod14/1 -> Mux/14
  "IW{1,1}(15,:)'"/1 -> dotprod15/1
  dotprod15/1 -> Mux/15
  "IW{1,1}(16,:)'"/1 -> dotprod16/1
  dotprod16/1 -> Mux/16
  "IW{1,1}(17,:)'"/1 -> dotprod17/1
  dotprod17/1 -> Mux/17
  "IW{1,1}(18,:)'"/1 -> dotprod18/1
  dotprod18/1 -> Mux/18
  "IW{1,1}(19,:)'"/1 -> dotprod19/1
  dotprod19/1 -> Mux/19
  "IW{1,1}(20,:)'"/1 -> dotprod20/1
  dotprod20/1 -> Mux/20
  "IW{1,1}(21,:)'"/1 -> dotprod21/1
  dotprod21/1 -> Mux/21
  "IW{1,1}(22,:)'"/1 -> dotprod22/1
  dotprod22/1 -> Mux/22
  "IW{1,1}(23,:)'"/1 -> dotprod23/1
  dotprod23/1 -> Mux/23
  "IW{1,1}(24,:)'"/1 -> dotprod24/1
  dotprod24/1 -> Mux/24
  "IW{1,1}(25,:)'"/1 -> dotprod25/1
  dotprod25/1 -> Mux/25
  "IW{1,1}(26,:)'"/1 -> dotprod26/1
  dotprod26/1 -> Mux/26
  "IW{1,1}(27,:)'"/1 -> dotprod27/1
  dotprod27/1 -> Mux/27
  "IW{1,1}(28,:)'"/1 -> dotprod28/1
  dotprod28/1 -> Mux/28
  "IW{1,1}(29,:)'"/1 -> dotprod29/1
  dotprod29/1 -> Mux/29
  "IW{1,1}(30,:)'"/1 -> dotprod30/1
  dotprod30/1 -> Mux/30
  Mux/1 -> "iz{1,1}"/1

== system mrefrobotarm_modified_previous_y_previous_u_previous_ref/const_51traces_30x30/Layer 2/Delays 1 ==
  "p{2}" : Inport  PortDimensions=30
      mask Display: e = 0.06;c1 = [120 230 180]/255;c2 = ([120 230 180]+0)/(256+128);c3 = ([120 230 180]+128)/(256+128);patch([0 1 1 0],[0 0 1 1],c1);patch([0 1 1 1-e 1-e 0+e],[0 0 1 1-e 0+e 0+e],c2);patch([0 0 1 1-e 0+e 0+e],[0 1 1 1-e 1-e 0+e],c3);plot([0 1 1 0 0],[0 0 1 1 0]);
  mux : Mux  Inputs=1
      mask Display: e = 0.06;c1 = [120 150 230]/255;c2 = ([120 150 230]+0)/383;c3 = ([120 150 230]+128)/383;patch([0 1 1 0],[0 0 1 1],c1);patch([0 1 1 1-e 1-e 0+e],[0 0 1 1-e 0+e 0+e],c2);patch([0 0 1 1-e 0+e 0+e],[0 1 1 1-e 1-e 0+e],c3);plot([0 1 1 0 0],[0 0 1 1 0]);disp('Mux')
  "pd{2,1}" : Outport
      mask Display: e = 0.06;c1 = [120 230 180]/255;c2 = ([120 230 180]+0)/(256+128);c3 = ([120 230 180]+128)/(256+128);patch([0 1 1 0],[0 0 1 1],c1);patch([0 1 1 1-e 1-e 0+e],[0 0 1 1-e 0+e 0+e],c2);patch([0 0 1 1-e 0+e 0+e],[0 1 1 1-e 1-e 0+e],c3);plot([0 1 1 0 0],[0 0 1 1 0]);
  wires:
  "p{2}"/1 -> mux/1
  mux/1 -> "pd{2,1}"/1
